simulink model "Problem2"  (R2018a)
settings: Solver=VariableStepAuto  StartTime=0.0  StopTime=10.0  RelTol=1e-3
values from neighbouring files (symbols this model uses):
  b = 0    [Problem2.m]    (also in Problem2Matlab.m = bv(4))
  J = 3    [Problem1.m]    (also in Problem2.m = 2; Problem2Matlab.m)
  k = 3    [Problem1.m]    (also in Problem2.m = 2; Problem2Matlab.m)
settings Model: Creator=User  LastModifiedBy=User

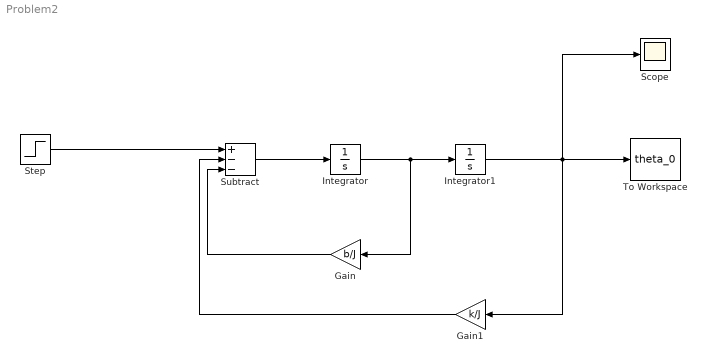
== system Problem2 ==
  Gain : Gain  Gain=b/J
  Gain1 : Gain  Gain=k/J
  Integrator : Integrator
  Integrator1 : Integrator
  Scope : Scope
  Step : Step  Time=0  SampleTime=0
  Subtract : Sum  Inputs=+--
  To Workspace : ToWorkspace  VariableName=theta_0  SampleTime=-1
      settings: Save2DSignal=2-D array (concatenate along first dimension)
  wires:
  Integrator/1 -> Integrator1/1, Gain/1
  Gain1/1 -> Subtract/2
  Gain/1 -> Subtract/3
  Subtract/1 -> Integrator/1
  Integrator1/1 -> Gain1/1, Scope/1, To Workspace/1
  Step/1 -> Subtract/1
